simulink model "without_in"  (R2018a)
settings: Solver=VariableStepAuto  StartTime=0.0  StopTime=30  RelTol=1e-3
settings Model: Creator=Halil Temurtaş  LastModifiedBy=Halil Temurtaş

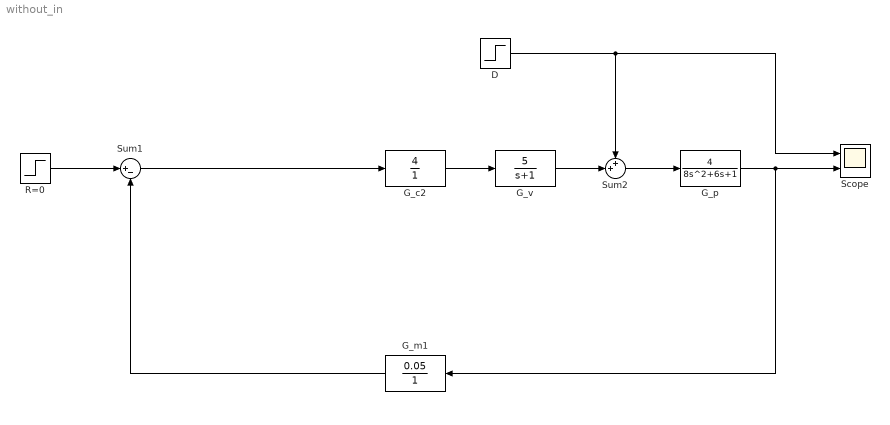
== system without_in ==
  D : Step  SampleTime=0
  G_c2 : TransferFcn  Numerator=[4]  Denominator=[1]
  G_m1 : TransferFcn  Numerator=[0.05]  Denominator=[1]
  G_p : TransferFcn  Numerator=[4]  Denominator=[8 6 1]
  G_v : TransferFcn  Numerator=[5]  Denominator=[1 1]
  R=0 : Step  After=0  SampleTime=0
  Scope : Scope  NumInputPorts=2
  Sum1 : Sum  Inputs=|+-
  Sum2 : Sum  Inputs=++|
  wires:
  G_v/1 -> Sum2/2
  G_c2/1 -> G_v/1
  Sum1/1 -> G_c2/1
  Sum2/1 -> G_p/1
  D/1 -> Sum2/1, Scope/1
  R=0/1 -> Sum1/1
  G_m1/1 -> Sum1/2
  G_p/1 -> Scope/2, G_m1/1
